simulink model "GFLIB_Asin_BAM"  (Simulink 7.3)
settings: Solver=ode45  StartTime=0.0  StopTime=10.0  RelTol=1e-3
settings Model: Creator=RE004C  LastModifiedBy=RE004C
settings HardwareCC: ProdIntDivRoundTo=Zero  ProdEndianess=BigEndian  ProdHWDeviceType=Freescale->32-bit PowerPC

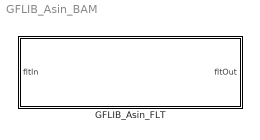
== system GFLIB_Asin_BAM ==
  GFLIB_Asin_FLT : Subsystem  mask(GFLIB_Asin_FLT){}
      mask help: Bit accurate model of GFLIB_Asin function, which computes the asin(fltIn) using the square based approximation.
      mask init:
      | pos = get_param(gcb, 'Position');width = pos(3) - pos(1); height = pos(4) - pos(2);tX=width/2;tY=height*0.9;
      mask Display: color('black');port_label('input',1,'fltIn');port_label('output',1,'fltOut');color('black');disp('GFLIB_Asin_FLT');color('blue');text(tX,tY, 'BAM', 'horizontalAlignment', 'center');

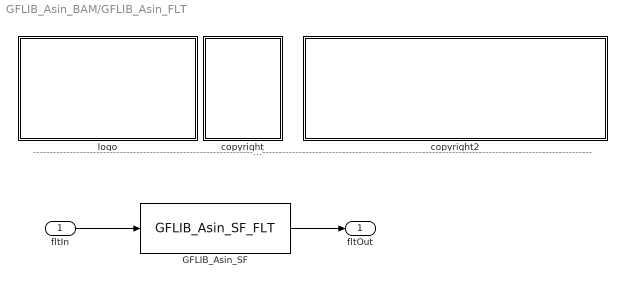
== system GFLIB_Asin_BAM/GFLIB_Asin_FLT ==
  note: ---------------------------------------------------------------------------------------------------------------------------------------------------------------------------------------------------
  fltIn : Inport  OutDataType=fixdt(1, 16)  OutScaling=2^0
  GFLIB_Asin_SF : S-Function  FunctionName=GFLIB_Asin_SF_FLT  EnableBusSupport=off
  copyright : Subsystem
      mask Display: text(10,90,'FILE:');text(10,75,'DESRIPTION:')text(10,60,'COPYRIGHT:')text(10,45,'VERSION:')text(10,30,'DATE:')
  copyright2 : Subsystem
      mask Display: text(10,90,'GFLIB_Asin_BAM_FLT.mdl');text(10,75,'Inverse cosine transformation');text(10,60,'Freescale')text(10,45,'0.1');text(10,30,'01-Sep-2011');
  logo : Subsystem
      mask Display: image(imread('logo.jpg'))
  fltOut : Outport  OutDataType=fixdt(1, 16)  OutScaling=2^0
  wires:
  fltIn/1 -> GFLIB_Asin_SF/1
  GFLIB_Asin_SF/1 -> fltOut/1

== system GFLIB_Asin_BAM/GFLIB_Asin_FLT/copyright ==

== system GFLIB_Asin_BAM/GFLIB_Asin_FLT/copyright2 ==

== system GFLIB_Asin_BAM/GFLIB_Asin_FLT/logo ==
